simulink model "chap17_4sim"  (Simulink 7.7)
settings: Solver=ode45  StartTime=0.0  StopTime=30  RelTol=1e-3
settings Model: Creator=ljk  LastModifiedBy=ljk
settings DataIOCC: SignalLoggingName=sigsOut
settings OptimizationCC: InitFltsAndDblsToZero=on
settings DebuggingCC: SaveWithParameterizedLinksMsg=none  SignalResolutionControl=TryResolveAllWithWarning  SolverPrmCheckMsg=none  MultiTaskDSMMsg=warning  MultiTaskCondExecSysMsg=none  StrictBusMsg=None
settings HardwareCC: TargetUnknown=on
settings RTWCC: IncludeERTFirstTime=on
settings GRTTargetCC: TargetFcnLib=ansi_tfl_tmw.mat

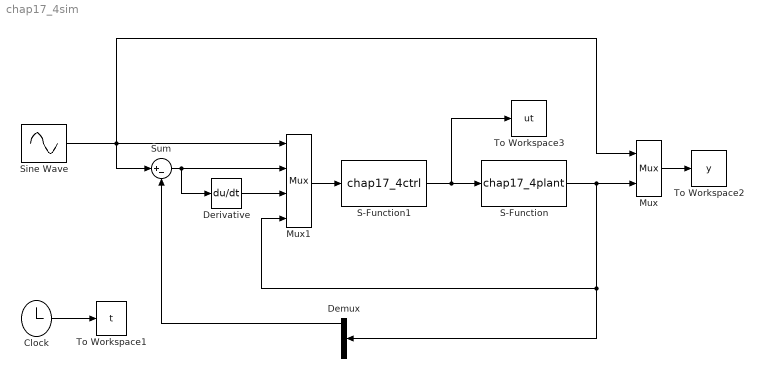
== system chap17_4sim ==
  Clock : Clock
      settings: Decimation=10
  Demux : Demux  Outputs=3
  Derivative : Derivative
  Mux : Mux  Inputs=2
  Mux1 : Mux
  S-Function : S-Function  FunctionName=chap17_4plant  EnableBusSupport=off
  S-Function1 : S-Function  FunctionName=chap17_4ctrl  EnableBusSupport=off
  Sine Wave : Sin  SampleTime=0
  Sum : Sum  Inputs=|+-  SaturateOnIntegerOverflow=on
  To Workspace1 : ToWorkspace  VariableName=t  SampleTime=-1  SaveFormat=Array
  To Workspace2 : ToWorkspace  VariableName=y  SampleTime=-1  SaveFormat=Array
  To Workspace3 : ToWorkspace  VariableName=ut  SampleTime=-1  SaveFormat=Array
  wires:
  Clock/1 -> To Workspace1/1
  Mux/1 -> To Workspace2/1
  Sine Wave/1 -> Mux1/1, Sum/1, Mux/1
  S-Function/1 -> Demux/1, Mux1/4, Mux/2
  S-Function1/1 -> S-Function/1, To Workspace3/1
  Demux/1 -> Sum/2
  Mux1/1 -> S-Function1/1
  Sum/1 -> Mux1/2, Derivative/1
  Derivative/1 -> Mux1/3
